simulink model "proj2"  (R2015a)
settings: Solver=ode45  StartTime=0.0  StopTime=10.0  RelTol=1e-3
values from neighbouring files (symbols this model uses):
  b = 200    [matlabparachot.mat]    (also in with_TF_1.m = 0.1)
  k1 = 226000    [matlabparachot.mat]
  k2 = 2325    [matlabparachot.mat]
  m1 = 40    [matlabparachot.mat]
  m2 = 416.5    [matlabparachot.mat]
libraries: fl_lib x10, nesl_utility x3
settings Model: Creator=ahmed alaa  LastModifiedBy=ahmed alaa

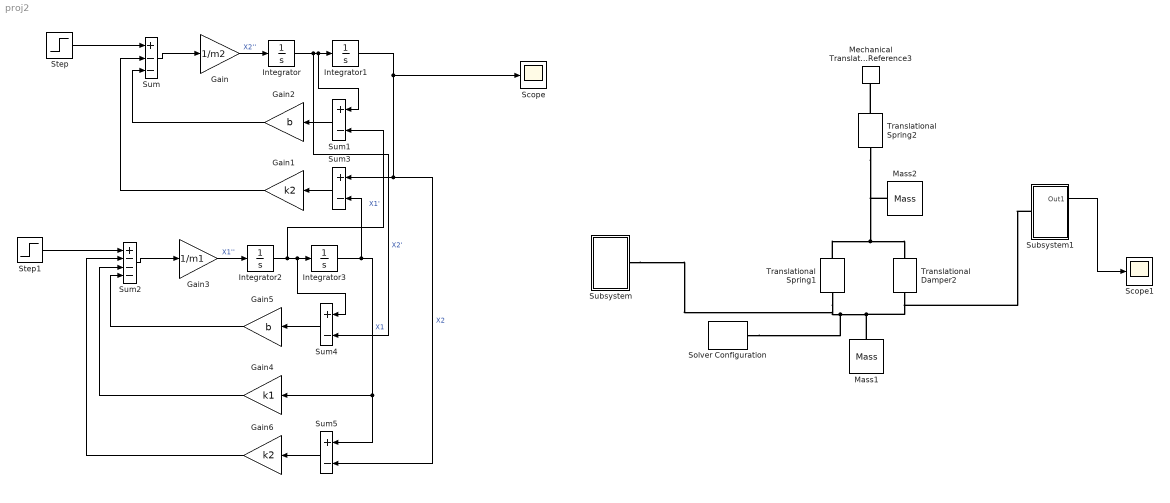
== system proj2 ==
  Gain : Gain  Gain=1/m2
  Gain1 : Gain  Gain=k2
  Gain2 : Gain  Gain=b
  Gain3 : Gain  Gain=1/m1
  Gain4 : Gain  Gain=k1
  Gain5 : Gain  Gain=b
  Gain6 : Gain  Gain=k2
  Integrator{,1..3} (4 alike) : Integrator
  Mass1 : fl_lib/Mechanical/Translational Elements/Mass  mass=m2 kg  v_specify=off  v_priority=High  v=0 m/s  f_specify=off  f_priority=High  f=0 N
  Mass2 : fl_lib/Mechanical/Translational Elements/Mass  mass=m1 kg  v_specify=off  v_priority=High  v=0 m/s  f_specify=off  f_priority=High  f=0 N
  Mechanical Translational Reference3 : fl_lib/Mechanical/Translational Elements/Mechanical Translational Reference
  Scope : Scope
      settings: YMin=-1  YMax=1
  Scope1 : Scope
      settings: TimeRange=60  YMin=0  YMax=10
  Solver Configuration : nesl_utility/Solver Configuration  PhysicalDomain=network_engine_domain  SubClassName=solver  LeftPortType=input  RightPortType=generic  Accelerate=off  Tones=[]  Harmonics=[]  SimulateNoise=off  Profile=off  UseLocalSampling=off  EnableSwitchedLinearOptims=on  FrequencyDomain=off  UseCCode=off  RelTol=0.001  AbsTol=1e-06  MinStep=1e-09  ToWorkspace=off  RevertToSquareIcSolve=off  NumHomotopyIterations=100  DoDC=off  ResidualTolerance=1e-09  UseLocalSolver=off  LocalSolverChoice=NE_BACKWARD_EULER_ADVANCER  LocalSolverSampleTime=0.001  DoFixedCost=off  MaxNonlinIter=3  MaxModeIter=2  LinearAlgebra=Sparse  DelaysMemoryBudget=1024  AutomaticFiltering=on  FilteringTimeConstant=0.001
  Step : Step  SampleTime=0
  Step1 : Step  SampleTime=0
  Subsystem : Subsystem
  Subsystem1 : Subsystem
  Sum : Sum  Inputs=+--
  Sum{1,3..5} (4 alike) : Sum  Inputs=+-
  Sum2 : Sum  Inputs=+---
  Translational Damper2 : fl_lib/Mechanical/Translational Elements/Translational Damper  D=b N/(m/s)  v_specify=off  v_priority=High  v=0 m/s  f_specify=off  f_priority=High  f=0 N
  Translational Spring1 : fl_lib/Mechanical/Translational Elements/Translational Spring  spr_rate=k2 N/m  v_specify=off  v_priority=High  v=0 m/s  f_specify=off  f_priority=High  f=0 N  x_specify=off  x_priority=High  x=0 m
  Translational Spring2 : fl_lib/Mechanical/Translational Elements/Translational Spring  spr_rate=k1 N/m  v_specify=off  v_priority=High  v=0 m/s  f_specify=off  f_priority=High  f=0 N  x_specify=off  x_priority=High  x=0 m
  wires:
  Integrator/1 -> Sum4/2, Sum1/1, Integrator1/1  "X2'"
  Integrator1/1 -> Sum5/2, Sum3/1, Scope/1  "X2"
  Gain/1 -> Integrator/1  "X2''"
  Sum/1 -> Gain/1
  Gain2/1 -> Sum/3
  Gain1/1 -> Sum/2
  Step/1 -> Sum/1
  Integrator2/1 -> Sum1/2, Sum4/1, Integrator3/1  "X1'"
  Integrator3/1 -> Sum3/2, Sum5/1, Gain4/1  "X1"
  Gain3/1 -> Integrator2/1  "X1''"
  Sum2/1 -> Gain3/1
  Gain5/1 -> Sum2/4
  Gain4/1 -> Sum2/3
  Step1/1 -> Sum2/1
  Sum1/1 -> Gain2/1
  Sum3/1 -> Gain1/1
  Sum4/1 -> Gain5/1
  Sum5/1 -> Gain6/1
  Gain6/1 -> Sum2/2
  Subsystem1/1(Out1) -> Scope1/1
  connections:
  Translational Spring1/LConn1 -- Mass2/LConn1 -- Translational Spring2/RConn1 -- Translational Damper2/LConn1
  Solver Configuration/RConn1 -- Subsystem/RConn1 -- Translational Spring1/RConn1 -- Subsystem1/LConn1 -- Translational Damper2/RConn1 -- Mass1/LConn1
  Translational Spring2/LConn1 -- Mechanical Translational Reference3/LConn1

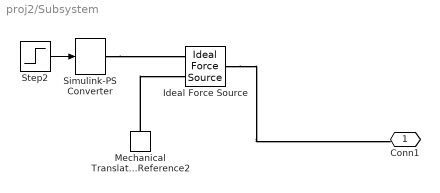
== system proj2/Subsystem ==
  Ideal Force Source : fl_lib/Mechanical/Mechanical Sources/Ideal Force Source
  Mechanical Translational Reference2 : fl_lib/Mechanical/Translational Elements/Mechanical Translational Reference
  Simulink-PS Converter : nesl_utility/Simulink-PS Converter  PhysicalDomain=network_engine_domain  SubClassName=ps_input  LeftPortType=input  RightPortType=output  PseudoPeriodic=off  Frequencies=[]  NoiseDistribution=none  NoiseParameters=[]  Unit=1  AffineConversion=off  InputFiltering=off  SimscapeFilterOrder=1  InputFilterTimeConstant=0.001  UdotUserProvided=1
  Step2 : Step  SampleTime=0
  Conn1 : PMIOPort  Port=1  Side=Right
  wires:
  Step2/1 -> Simulink-PS Converter/1
  connections:
  Ideal Force Source/LConn1 -- Conn1/RConn1
  Mechanical Translational Reference2/LConn1 -- Ideal Force Source/RConn2
  Simulink-PS Converter/RConn1 -- Ideal Force Source/RConn1

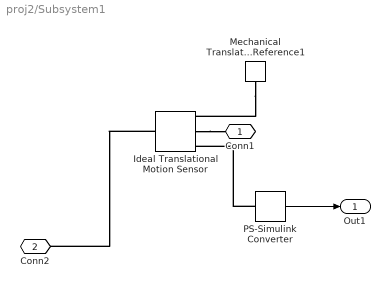
== system proj2/Subsystem1 ==
  Ideal Translational Motion Sensor : fl_lib/Mechanical/Mechanical Sensors/Ideal Translational Motion Sensor  offset=0 m
  Mechanical Translational Reference1 : fl_lib/Mechanical/Translational Elements/Mechanical Translational Reference
  PS-Simulink Converter : nesl_utility/PS-Simulink Converter  PhysicalDomain=network_engine_domain  SubClassName=ps_output  LeftPortType=input  RightPortType=output  PseudoPeriodic=off  Frequencies=[]  Unit=1  AffineConversion=off
  Conn1 : PMIOPort  Port=1  Side=Right
  Conn2 : PMIOPort  Port=2  Side=Left
  Out1 : Outport
  wires:
  PS-Simulink Converter/1 -> Out1/1
  connections:
  Ideal Translational Motion Sensor/RConn2 -- Conn1/RConn1
  Ideal Translational Motion Sensor/LConn1 -- Conn2/RConn1
  Mechanical Translational Reference1/LConn1 -- Ideal Translational Motion Sensor/RConn1
  PS-Simulink Converter/LConn1 -- Ideal Translational Motion Sensor/RConn3
